simulink model "load_from_files_1_sm_master"  (R2021b)
settings: Solver=ode4  StartTime=0.0  StopTime=inf  FixedStep=0.001  RelTol=1e-3  EnableMultiTasking=on
model workspace (MATLAB code in the model file):
  | % Add the class folders into the path.
  | addpath src\model
  | addpath src\utils
  | 
  | %% Loading data from files.
  | % Data for supervisor 1.
  | utils = StateMachineUtils;
  | 
  | % From TCT: Load all events' number.
  | utils = utils.loadEventsInAds('resources/tct/ALLEVENT.ADS');
  | 
  | % From TCT: Disabled events in each state.
  | utils = utils.loadDisabledEventsInPdt('resources/tct/supervisor1/DATA_SIMSUP1_MG1.PDT');
  | 
  | % From TCT: Transition matrix.
  | utils = utils.loadTransitionsInAds('resources/tct/supervisor1/SIMSUP1_MG1.ADS');
  | 
  | % Parameters for the block.
  | encodedStates = StateEncoder.encode(utils.statesArray);
  | 
  | transitions = utils.transitions;
  | 
  | allEvents = utils.eventsArray;
libraries: opal_lib x3
Description:
  | Model of a simple control system for use iin training.
settings Model: Creator=Paul Baracos  LastModifiedBy=andrerangel
settings SolverCC: AlgebraicLoopSolver=TrustRegion
settings DataIOCC: LimitDataPoints=on  SaveFormat=Array  SignalLoggingSaveFormat=ModelDataLogs  SaveOutput=off  SaveTime=off  ReturnWorkspaceOutputs=off  SignalLoggingName=sigsOut
settings OptimizationCC: BlockReduction=off  BooleanDataType=off  OptimizeBlockIOStorage=off  BufferReuse=off  ExpressionFolding=off  LocalBlockOutputs=off  InitFltsAndDblsToZero=on  LifeSpan=inf
settings DebuggingCC: SaveWithParameterizedLinksMsg=none  UnderspecifiedInitializationDetection=Classic  MergeDetectMultiDrivingBlocksExec=none  SignalResolutionControl=TryResolveAllWithWarning  MultiTaskDSMMsg=warning  MultiTaskCondExecSysMsg=none  FcnCallInpInsideContextMsg=warning  SFUnexpectedBacktrackingDiag=warning  SFNoUnconditionalDefaultTransitionDiag=warning  SFExecutionAtInitializationDiag=none  SFMachineParentedDataDiag=warning  ArithmeticOperatorsInVariantConditions=warning
settings HardwareCC: ProdBitPerPointer=32  ProdBitPerSizeT=32  ProdBitPerPtrDiffT=32  ProdLargestAtomicFloat=None  ProdIntDivRoundTo=Undefined  ProdEndianess=Unspecified  ProdWordSize=32  ProdHWDeviceType=32-bit Generic  TargetUnknown=on
settings ModelReferenceCC: PropagateSignalLabelsOutOfModel=off
settings SFSimCC: SimUseLocalCustomCode=off  CustomCodeUndefinedFunction=UseInterfaceOnly
settings RTWCC: GenCodeOnly=on  RTWUseLocalCustomCode=off
settings CodeAppCC: StateflowObjectComments=on
settings GRTTargetCC: TargetFcnLib=ansi_tfl_tmw.mat  TargetLangStandard=C89/C90 (ANSI)  CombineOutputUpdateFcns=off  GRTInterface=on
settings ConfigComp: CovMetricSettings=dw  CovSaveCumulativeToWorkspaceVar=on  CovSaveSingleToWorkspaceVar=on  CovExternalEMLEnable=off

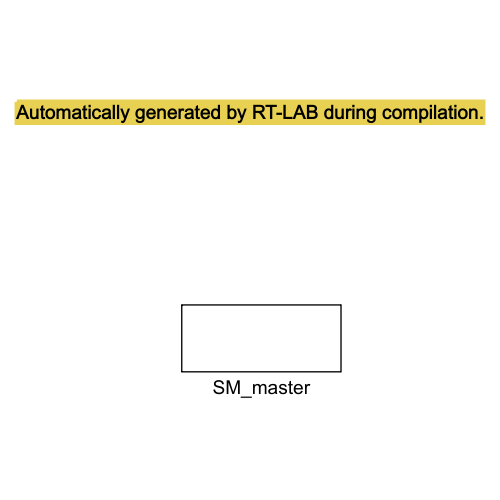
[thumbnail: Simulink's stored preview of the top-level diagram]
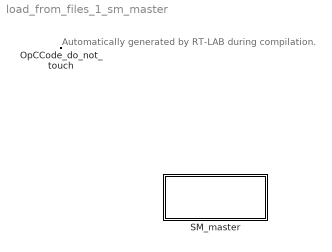
== system load_from_files_1_sm_master ==
  note: Automatically generated by RT-LAB during compilation.
  OpCCode_do_not_touch : opal_lib/Communication/OpCCode  SystemSampleTime=-1  VariantActivationTime=update diagram  Latency=0  AutoFrameSizeCalculation=off
  SM_master : Subsystem

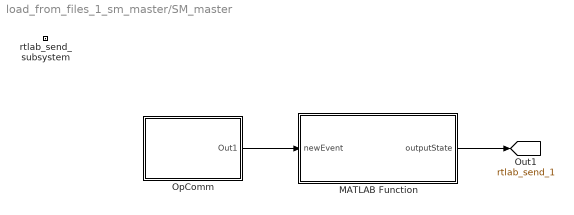
== system load_from_files_1_sm_master/SM_master ==
  MATLAB Function : MATLAB Function  TreatAsAtomicUnit=on
  OpComm : Subsystem
      mask init:
      | opmaskdisplay('maskdisplay_block',gcb,'disp(''OpComm'')');
      mask Display:
      | patch([0 0.5 0.7 0],[1 1 0 0],[0.7 0.75 0.9]);
      | patch([1 0.53 0.73 1],[1 1 0 0],[1 0.8 0.7]);
      | plot([0 0 1 1 0],[0 1 1 0 0]);
      | disp('OpComm')
  rtlab_send_subsystem : Subsystem  Priority=-100
      mask Display: text(0,0,'');
  tag scope: rtlab_send_1=global
  wires:
  OpComm/1(Out1) -> MATLAB Function/1(newEvent)
  MATLAB Function/1(outputState) -> [rtlab_send_1]

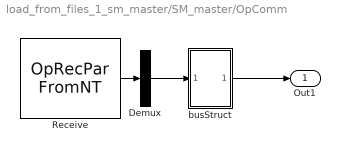
== system load_from_files_1_sm_master/SM_master/OpComm ==
  Demux : Demux  Outputs=[1]
  Receive : opal_lib/Communication/OpRecPar FromNT  Data_width=1  InitialConditions=11
  busStruct : Subsystem
  Out1 : Outport
  wires:
  Demux/1 -> busStruct/1(In1)
  busStruct/1(Out1) -> Out1/1
  Receive/1 -> Demux/1

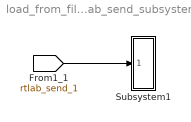
== system load_from_files_1_sm_master/SM_master/rtlab_send_subsystem ==
  Subsystem1 : Subsystem
  wires:
  [rtlab_send_1] -> Subsystem1/1(In1)

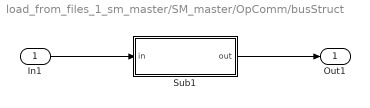
== system load_from_files_1_sm_master/SM_master/OpComm/busStruct ==
  In1 : Inport
  Sub1 : Subsystem
  Out1 : Outport
  wires:
  Sub1/1(out) -> Out1/1
  In1/1 -> Sub1/1(in)

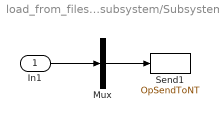
== system load_from_files_1_sm_master/SM_master/rtlab_send_subsystem/Subsystem1 ==
  In1 : Inport
  Mux : Mux  Inputs=1
  Send1 : opal_lib/Communication/OpSendToNT  Acqu_group=1
  wires:
  Mux/1 -> Send1/1
  In1/1 -> Mux/1

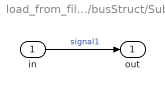
== system load_from_files_1_sm_master/SM_master/OpComm/busStruct/Sub1 ==
  in : Inport
  out : Outport
  wires:
  in/1 -> out/1  "signal1"

== matlab function load_from_files_1_sm_master/SM_master/MATLAB Function ==
  data: newEvent input; outputState output; allEvents parameter; transitions parameter; encodedStates parameter
function outputState  = stateMachine(newEvent, allEvents, transitions, encodedStates)
% State Machine with parameters from files.

% Initialize a persistent object. Its value will not be erased as this
% block finishes.
persistent stateMachine

% Assign the persistent object to the StateMachine class with data passed
% as parameters.
if (isempty(stateMachine))
    statesArray = StateEncoder.decode(encodedStates);                        
    stateMachine = StateMachine(statesArray, transitions, allEvents);
end

stateMachine.inputEvent = newEvent;
outputState = double(stateMachine.currentState.number);
% isActiveArray = stateMachine.currentState.activeEvents;
% eventsNumber = stateMachine.eventsArray;
